simulink model "zad2"  (R2025b)
settings: Solver=VariableStepAuto  StartTime=0.0  StopTime=3500  RelTol=1e-3
libraries: fuzblock x2
settings Model: Creator=jovan  LastModifiedBy=Katarina

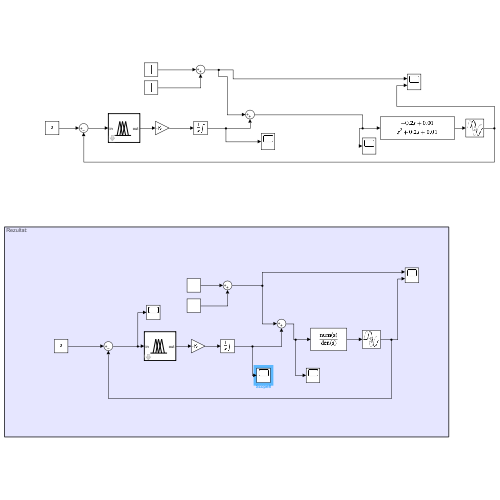
[thumbnail: Simulink's stored preview of the top-level diagram]
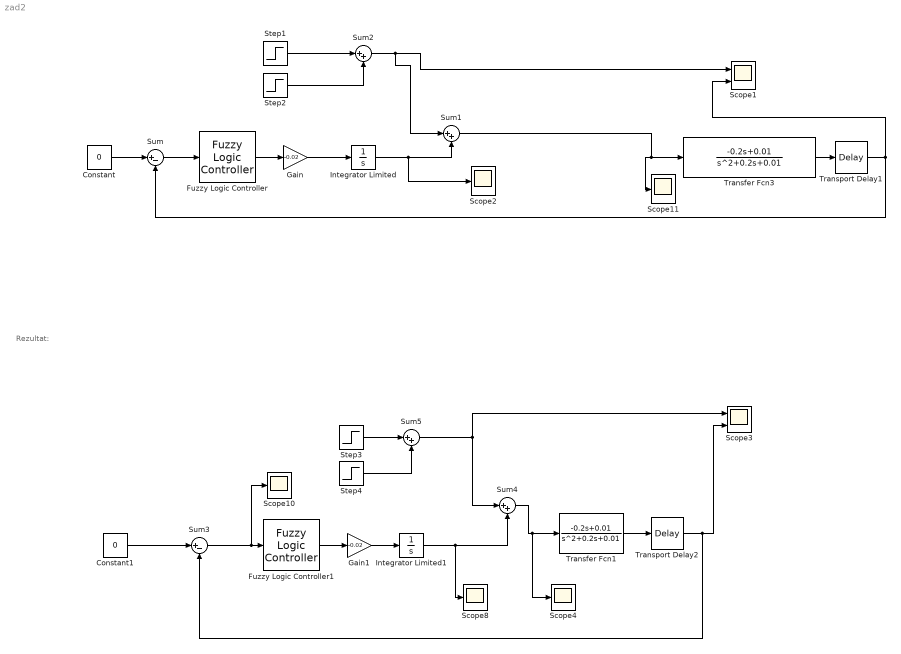
== system zad2 ==
  note: Rezultat:
  Constant : Constant  Value=0
  Constant1 : Constant  Value=0
  Fuzzy Logic Controller : fuzblock/Fuzzy Logic  Controller  FIS='kontrolaBrzine.fis'  OutputSampleNumber=101  DataType=double  UseLookupTable=off  NumBreakpoints=10  FuzzifiedInputs=off  RuleFiringStrengths=off  RuleOutputs=off  AggregatedOutputs=off  SimulateUsing=Interpreted execution  OutOfRangeInputValueMessage=warning  NoRuleFiredMessage=warning  EmptyOutputFuzzySetMessage=warning
  Fuzzy Logic Controller1 : fuzblock/Fuzzy Logic  Controller  FIS='kontrolaBrzineV2.fis'  OutputSampleNumber=101  DataType=double  UseLookupTable=off  NumBreakpoints=10  FuzzifiedInputs=off  RuleFiringStrengths=off  RuleOutputs=off  AggregatedOutputs=off  SimulateUsing=Interpreted execution  OutOfRangeInputValueMessage=warning  NoRuleFiredMessage=warning  EmptyOutputFuzzySetMessage=warning
  Gain : Gain  Gain=-0.02
  Gain1 : Gain  Gain=-0.02
  Integrator Limited : Integrator  LimitOutput=on  UpperSaturationLimit=0.75  LowerSaturationLimit=-0.75
  Integrator Limited1 : Integrator  LimitOutput=on  UpperSaturationLimit=0.75  LowerSaturationLimit=-0.75
  Scope1 : Scope  NumInputPorts=2
      settings: ActiveDisplayYMinimum=-1.461911168167181  ActiveDisplayYMaximum=2.2253042357482924
  Scope{2,4,8,10..11} (5 alike) : Scope
      Scope10 settings: ActiveDisplayYMinimum=-1.3140352599112908  ActiveDisplayYMaximum=1.7899467543150394  DataLoggingVariableName=ScopeData2
      Scope11 settings: ActiveDisplayYMinimum=-1.7304588396468332  ActiveDisplayYMaximum=2.1411173344644125  DataLoggingVariableName=ScopeData10
      Scope2 settings: ActiveDisplayYMinimum=-1.9808295586445803  ActiveDisplayYMaximum=0.58677789667896685
      Scope4 settings: ActiveDisplayYMinimum=-1  ActiveDisplayYMaximum=1  DataLoggingVariableName=ScopeData7
      Scope8 settings: ActiveDisplayYMinimum=-0.69092946920040377  ActiveDisplayYMaximum=0.93773596491271893  DataLoggingVariableName=ScopeData9
  Scope3 : Scope  NumInputPorts=2
      settings: ActiveDisplayYMinimum=-2.4101026727885233  ActiveDisplayYMaximum=1.4575508245182593  DataLoggingVariableName=ScopeData3
  Step1 : Step  Time=1000  After=0.75  SampleTime=0
  Step2 : Step  Time=2000  After=-0.75  SampleTime=0
  Step3 : Step  Time=1000  After=0.75  SampleTime=0
  Step4 : Step  Time=2000  After=-0.75  SampleTime=0
  Sum : Sum  Inputs=|+-
  Sum{1..2,4..5} (4 alike) : Sum  Inputs=|++
  Sum3 : Sum  Inputs=|+-
  Transfer Fcn1 : TransferFcn  Numerator=[-0.2 0.01]  Denominator=[1 0.2 0.01]
  Transfer Fcn3 : TransferFcn  Numerator=[-0.2 0.01]  Denominator=[1 0.2 0.01]
  Transport Delay1 : TransportDelay  DelayTime=4
  Transport Delay2 : TransportDelay  DelayTime=4
  wires:
  Sum1/1 -> Transfer Fcn3/1, Scope11/1
  Step2/1 -> Sum2/2
  Sum/1 -> Fuzzy Logic Controller/1
  Constant/1 -> Sum/1
  Sum2/1 -> Sum1/1, Scope1/1
  Step1/1 -> Sum2/1
  Transfer Fcn3/1 -> Transport Delay1/1
  Transport Delay1/1 -> Scope1/2, Sum/2
  Sum5/1 -> Sum4/1, Scope3/1
  Sum4/1 -> Scope4/1, Transfer Fcn1/1
  Step4/1 -> Sum5/2
  Transfer Fcn1/1 -> Transport Delay2/1
  Sum3/1 -> Scope10/1, Fuzzy Logic Controller1/1
  Transport Delay2/1 -> Scope3/2, Sum3/2
  Step3/1 -> Sum5/1
  Constant1/1 -> Sum3/1
  Gain/1 -> Integrator Limited/1
  Fuzzy Logic Controller/1 -> Gain/1
  Integrator Limited/1 -> Scope2/1, Sum1/2
  Gain1/1 -> Integrator Limited1/1
  Fuzzy Logic Controller1/1 -> Gain1/1
  Integrator Limited1/1 -> Sum4/2, Scope8/1
